simulink model "ball_on_beam"  (R2020a)
settings: Solver=VariableStepAuto  StartTime=0.0  StopTime=100.0  RelTol=1e-3
settings Model: Creator=emile  LastModifiedBy=emile

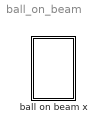
== system ball_on_beam ==
  ball on beam x : Subsystem

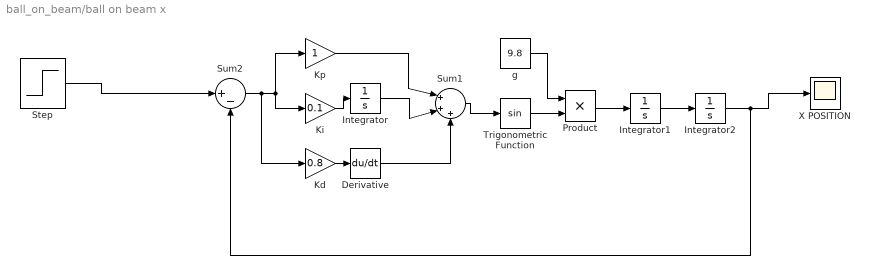
== system ball_on_beam/ball on beam x ==
  Derivative : Derivative
  Integrator : Integrator
  Integrator1 : Integrator
  Integrator2 : Integrator
  Kd : Gain  Gain=0.8
  Ki : Gain  Gain=0.1
  Kp : Gain
  Product : Product
  Step : Step  After=2  SampleTime=0.1
  Sum1 : Sum  Inputs=|+++
  Sum2 : Sum  Inputs=|+-
  Trigonometric Function : Trigonometry
  X POSITION : Scope
  g : Constant  Value=9.8
  wires:
  g/1 -> Product/1
  Product/1 -> Integrator1/1
  Integrator1/1 -> Integrator2/1
  Integrator2/1 -> Sum2/2, X POSITION/1
  Ki/1 -> Integrator/1
  Step/1 -> Sum2/1
  Kd/1 -> Derivative/1
  Kp/1 -> Sum1/1
  Integrator/1 -> Sum1/2
  Derivative/1 -> Sum1/3
  Sum1/1 -> Trigonometric Function/1
  Sum2/1 -> Kd/1, Ki/1, Kp/1
  Trigonometric Function/1 -> Product/2
